simulink model "sim_IntMRE_case3"  (R2023a)
settings: Solver=ode3  StartTime=0.0  StopTime=150  FixedStep=Ts  MaxStep=Ts  RelTol=1e-4
values from neighbouring files (symbols this model uses):
  b0 = 30    [Initial_par.m]
  b1 = 11    [Initial_par.m]
  c1 = 1    [Initial_par.m]    (also in Regressor.m = c(1); virtual_ctrl.m = c(1))
  c2 = 1    [Initial_par.m]    (also in Regressor.m = c(2); virtual_ctrl.m = c(2))
  c3 = 1    [Initial_par.m]    (also in Regressor.m = c(3); virtual_ctrl.m = c(3))
  gamma = 10    [Initial_par.m]
  kpa = [kap1,kap2,kap3]    [Initial_par.m]
  N = 3    [Initial_par.m]
  tau_d = 5    [Initial_par.m]
  th = [0.4,0.5,0.1]'    [Initial_par.m]    (also in Regressor.m = th_ext(:,1); virtual_ctrl.m = th_ext(:,1))
  Ts = 1e-3    (= 0.001)    [Initial_par.m]
  vari = SD^2    (= 1e-08)    [Initial_par.m]
  x0 = [0,0,0]'    [Initial_par.m]    (also in TO_sys.m = x_init)
  zeta0 = -z0    [Initial_par.m]
undefined symbols (not defined in the file or in its folder): Phi0, z0
libraries: matrix_library x6
settings Model: Creator=stt  LastModifiedBy=stt
settings SolverCC: SolverResetMethod=Robust
settings OptimizationCC: ReuseModelBlockBuffer=off

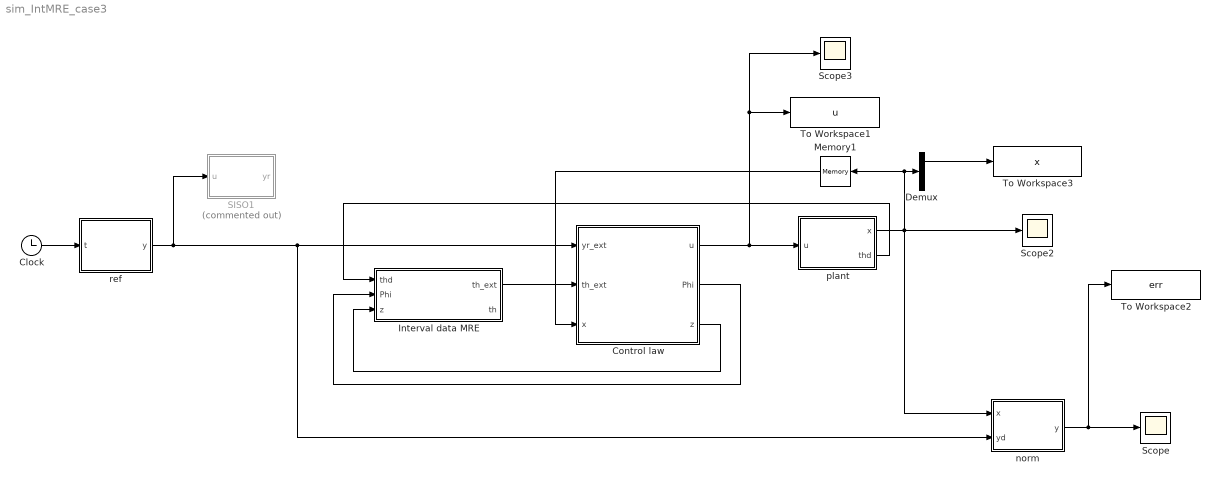
== system sim_IntMRE_case3 ==
  Clock : Clock
  Control law : Subsystem
  Demux : Demux  Outputs=3
  Interval data MRE : Subsystem
  Memory1 : Memory  InitialCondition=x0
  SISO1 : Subsystem  Commented=on
  Scope : Scope
  Scope2 : Scope
  Scope3 : Scope
  To Workspace1 : ToWorkspace  VariableName=u  SaveFormat=Timeseries  SampleTime=-1
  To Workspace2 : ToWorkspace  VariableName=err  SaveFormat=Timeseries  SampleTime=-1
  To Workspace3 : ToWorkspace  VariableName=x  SaveFormat=Timeseries  SampleTime=-1
  norm : MATLAB Function  TreatAsAtomicUnit=on
  plant : Subsystem
  ref : MATLAB Function  TreatAsAtomicUnit=on
  wires:
  ref/1(y) -> norm/2(yd), Control law/1(yr_ext), SISO1/1(u)
  norm/1(y) -> To Workspace2/1, Scope/1
  plant/1(x) -> Demux/1, Memory1/1, norm/1(x), Scope2/1
  Demux/1 -> To Workspace3/1
  Clock/1 -> ref/1(t)
  Control law/2(Phi) -> Interval data MRE/2(Phi)
  Control law/1(u) -> To Workspace1/1, Scope3/1, plant/1(u)
  Memory1/1 -> Control law/3(x)
  Interval data MRE/1(th_ext) -> Control law/2(th_ext)
  Control law/3(z) -> Interval data MRE/3(z)
  plant/2(thd) -> Interval data MRE/1(thd)

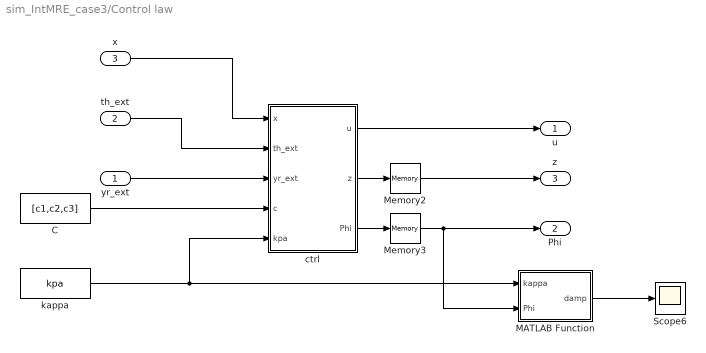
== system sim_IntMRE_case3/Control law ==
  yr_ext : Inport
  th_ext : Inport  Port=2
  x : Inport  Port=3
  C : Constant  Value=[c1,c2,c3]
  MATLAB Function : MATLAB Function  TreatAsAtomicUnit=on
  Memory2 : Memory  InitialCondition=z0
  Memory3 : Memory  InitialCondition=Phi0
  Scope6 : Scope
  ctrl : MATLAB Function  TreatAsAtomicUnit=on
  kappa : Constant  Value=kpa
  u : Outport
  Phi : Outport  Port=2
  z : Outport  Port=3
  wires:
  ctrl/3(Phi) -> Memory3/1
  Memory3/1 -> MATLAB Function/2(Phi), Phi/1
  th_ext/1 -> ctrl/2(th_ext)
  kappa/1 -> ctrl/5(kpa), MATLAB Function/1(kappa)
  C/1 -> ctrl/4(c)
  Memory2/1 -> z/1
  ctrl/2(z) -> Memory2/1
  yr_ext/1 -> ctrl/3(yr_ext)
  x/1 -> ctrl/1(x)
  ctrl/1(u) -> u/1
  MATLAB Function/1(damp) -> Scope6/1

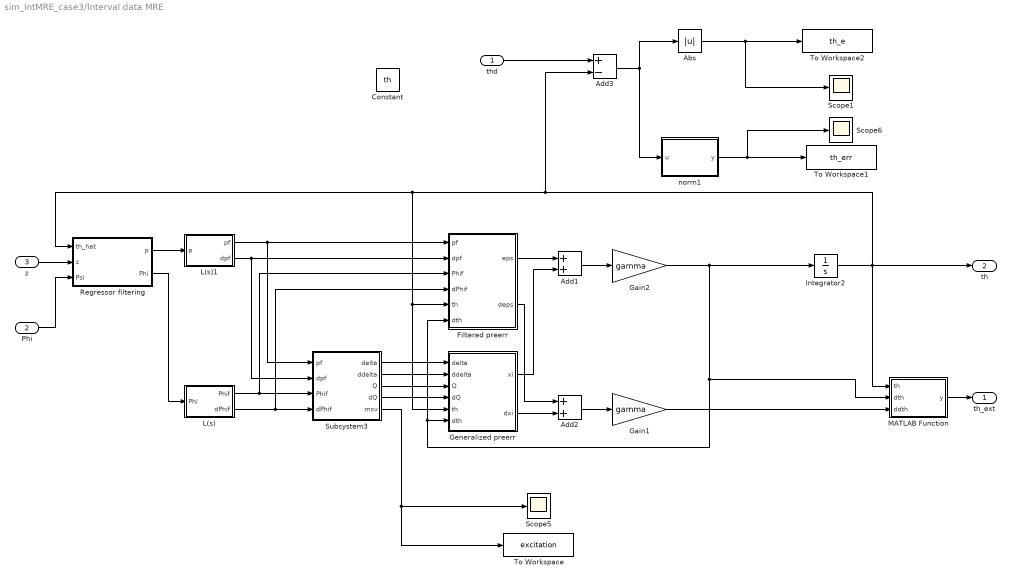
== system sim_IntMRE_case3/Interval data MRE ==
  thd : Inport
  Phi : Inport  Port=2
  z : Inport  Port=3
  Abs : Abs  SaturateOnIntegerOverflow=off
  Add1 : Sum
  Add2 : Sum
  Add3 : Sum  Inputs=+-
  Constant : Constant  Value=th
  Filtered preerr : Subsystem
  Gain1 : Gain  Gain=gamma
  Gain2 : Gain  Gain=gamma
  Generalized preerr : Subsystem
  Integrator2 : Integrator  InitialCondition=zeros(N,1)
  L(s) : Subsystem
  L(s)1 : Subsystem
  MATLAB Function : MATLAB Function  TreatAsAtomicUnit=on
  Regressor filtering : Subsystem
  Scope1 : Scope
  Scope5 : Scope
  Scope6 : Scope
  Subsystem3 : Subsystem
  To Workspace : ToWorkspace  VariableName=excitation  SaveFormat=Timeseries  SampleTime=-1
  To Workspace1 : ToWorkspace  VariableName=th_err  SaveFormat=Timeseries  SampleTime=-1
  To Workspace2 : ToWorkspace  VariableName=th_e  SaveFormat=Timeseries  SampleTime=-1
  norm1 : MATLAB Function  TreatAsAtomicUnit=on
  th_ext : Outport
  th : Outport  Port=2
  wires:
  MATLAB Function/1(y) -> th_ext/1
  norm1/1(y) -> To Workspace1/1, Scope6/1
  thd/1 -> Add3/1
  Regressor filtering/2(Phi) -> L(s)/1(Phi)
  Regressor filtering/1(p) -> L(s)1/1(p)
  z/1 -> Regressor filtering/2(z)
  Phi/1 -> Regressor filtering/3(Psi)
  Integrator2/1 -> MATLAB Function/1(th), th/1, Generalized preerr/5(th), Filtered preerr/5(th), Regressor filtering/1(th_hat), Add3/2
  Add3/1 -> norm1/1(u), Abs/1
  Abs/1 -> To Workspace2/1, Scope1/1
  L(s)1/1(pf) -> Filtered preerr/1(pf), Subsystem3/1(pf)
  L(s)1/2(dpf) -> Subsystem3/2(dpf), Filtered preerr/2(dpf)
  L(s)/1(Phif) -> Filtered preerr/3(Phif), Subsystem3/3(Phif)
  L(s)/2(dPhif) -> Filtered preerr/4(dPhif), Subsystem3/4(dPhif)
  Subsystem3/2(ddelta) -> Generalized preerr/2(ddelta)
  Subsystem3/3(Q) -> Generalized preerr/3(Q)
  Subsystem3/4(dQ) -> Generalized preerr/4(dQ)
  Subsystem3/5(msv) -> To Workspace/1, Scope5/1
  Subsystem3/1(delta) -> Generalized preerr/1(delta)
  Gain1/1 -> MATLAB Function/3(ddth)
  Add1/1 -> Gain2/1
  Filtered preerr/1(eps) -> Add1/1
  Generalized preerr/1(xi) -> Add1/2
  Generalized preerr/2(dxi) -> Add2/2
  Add2/1 -> Gain1/1
  Filtered preerr/2(deps) -> Add2/1
  Gain2/1 -> Filtered preerr/6(dth), Generalized preerr/6(dth), MATLAB Function/2(dth), Integrator2/1

== system sim_IntMRE_case3/SISO1 ==
  u : Inport
  Mux : Mux
  Scope3 : Scope
  Transfer Fcn : TransferFcn  Numerator=[16]  Denominator=[1 8 24 32 16]
  Transfer Fcn1 : TransferFcn  Numerator=[16 0]  Denominator=[1 8 24 32 16]
  Transfer Fcn2 : TransferFcn  Numerator=[16 0 0]  Denominator=[1 8 24 32 16]
  Transfer Fcn3 : TransferFcn  Numerator=[16 0 0 0]  Denominator=[1 8 24 32 16]
  yr : Outport
  wires:
  u/1 -> Transfer Fcn3/1, Transfer Fcn2/1, Transfer Fcn1/1, Transfer Fcn/1
  Transfer Fcn/1 -> Scope3/1, Mux/1
  Transfer Fcn1/1 -> Mux/2
  Transfer Fcn2/1 -> Mux/3
  Transfer Fcn3/1 -> Mux/4
  Mux/1 -> yr/1

== system sim_IntMRE_case3/plant ==
  u : Inport
  Add : Sum
  MATLAB Function : MATLAB Function  TreatAsAtomicUnit=on
  Random Number : RandomNumber  Variance=vari  SampleTime=Ts
  S-Function : S-Function  FunctionName=TO_sys  Parameters=x0,th  SFunctionDeploymentMode=off  EnableBusSupport=off
  x : Outport
  thd : Outport  Port=2
  wires:
  u/1 -> S-Function/1
  S-Function/1 -> MATLAB Function/1(u)
  Add/1 -> x/1
  MATLAB Function/2(thd) -> thd/1
  MATLAB Function/1(x) -> Add/2

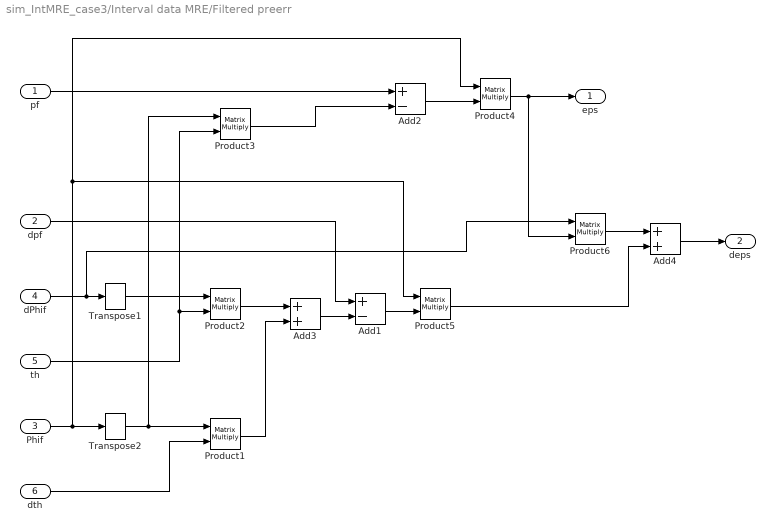
== system sim_IntMRE_case3/Interval data MRE/Filtered preerr ==
  pf : Inport
  dpf : Inport  Port=2
  Phif : Inport  Port=3
  dPhif : Inport  Port=4
  th : Inport  Port=5
  dth : Inport  Port=6
  Add1 : Sum  Inputs=+-
  Add2 : Sum  Inputs=+-
  Add3 : Sum
  Add4 : Sum
  Product{1..6} (6 alike) : Product  Multiplication=Matrix(*)
  Transpose1 : matrix_library/Transpose
  Transpose2 : matrix_library/Transpose
  eps : Outport
  deps : Outport  Port=2
  wires:
  Product2/1 -> Add3/1
  Phif/1 -> Product4/1, Product5/1, Transpose2/1
  dth/1 -> Product1/2
  Product1/1 -> Add3/2
  Add3/1 -> Add1/2
  dpf/1 -> Add1/1
  th/1 -> Product3/2, Product2/2
  Product3/1 -> Add2/2
  Transpose2/1 -> Product3/1, Product1/1
  pf/1 -> Add2/1
  Product4/1 -> Product6/2, eps/1
  Transpose1/1 -> Product2/1
  Add4/1 -> deps/1
  Add2/1 -> Product4/2
  Add1/1 -> Product5/2
  Product5/1 -> Add4/2
  dPhif/1 -> Product6/1, Transpose1/1
  Product6/1 -> Add4/1

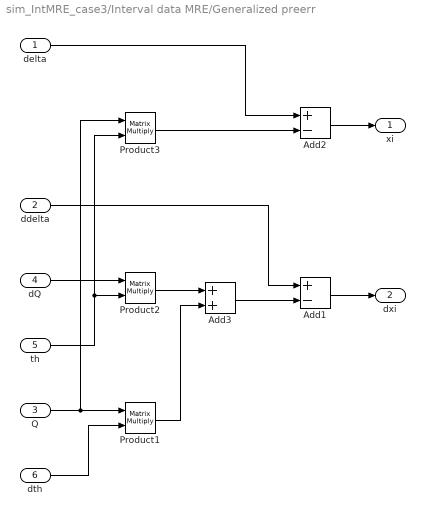
== system sim_IntMRE_case3/Interval data MRE/Generalized preerr ==
  delta : Inport
  ddelta : Inport  Port=2
  Q : Inport  Port=3
  dQ : Inport  Port=4
  th : Inport  Port=5
  dth : Inport  Port=6
  Add1 : Sum  Inputs=+-
  Add2 : Sum  Inputs=+-
  Add3 : Sum
  Product1 : Product  Multiplication=Matrix(*)
  Product2 : Product  Multiplication=Matrix(*)
  Product3 : Product  Multiplication=Matrix(*)
  xi : Outport
  dxi : Outport  Port=2
  wires:
  dQ/1 -> Product2/1
  Product2/1 -> Add3/1
  dth/1 -> Product1/2
  Product1/1 -> Add3/2
  Add3/1 -> Add1/2
  ddelta/1 -> Add1/1
  Add1/1 -> dxi/1
  th/1 -> Product3/2, Product2/2
  Product3/1 -> Add2/2
  Q/1 -> Product3/1, Product1/1
  delta/1 -> Add2/1
  Add2/1 -> xi/1

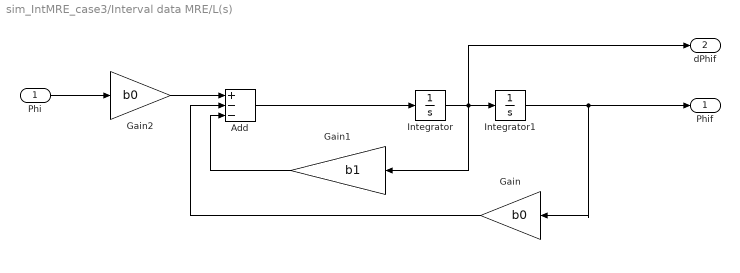
== system sim_IntMRE_case3/Interval data MRE/L(s) ==
  Phi : Inport
  Add : Sum  Inputs=+--
  Gain : Gain  Gain=b0
  Gain1 : Gain  Gain=b1
  Gain2 : Gain  Gain=b0
  Integrator : Integrator
  Integrator1 : Integrator
  Phif : Outport
  dPhif : Outport  Port=2
  wires:
  Phi/1 -> Gain2/1
  Integrator1/1 -> Gain/1, Phif/1
  Add/1 -> Integrator/1
  Integrator/1 -> Gain1/1, dPhif/1, Integrator1/1
  Gain1/1 -> Add/3
  Gain/1 -> Add/2
  Gain2/1 -> Add/1

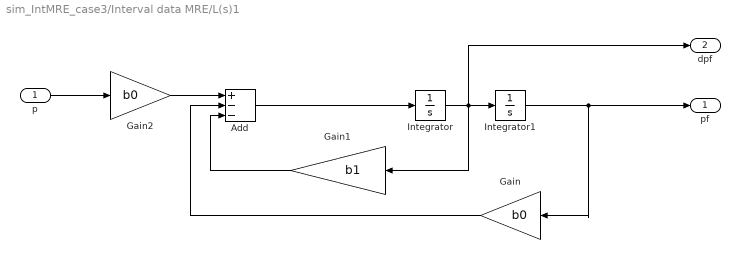
== system sim_IntMRE_case3/Interval data MRE/L(s)1 ==
  p : Inport
  Add : Sum  Inputs=+--
  Gain : Gain  Gain=b0
  Gain1 : Gain  Gain=b1
  Gain2 : Gain  Gain=b0
  Integrator : Integrator
  Integrator1 : Integrator
  pf : Outport
  dpf : Outport  Port=2
  wires:
  p/1 -> Gain2/1
  Integrator1/1 -> Gain/1, pf/1
  Add/1 -> Integrator/1
  Integrator/1 -> Gain1/1, dpf/1, Integrator1/1
  Gain1/1 -> Add/3
  Gain/1 -> Add/2
  Gain2/1 -> Add/1

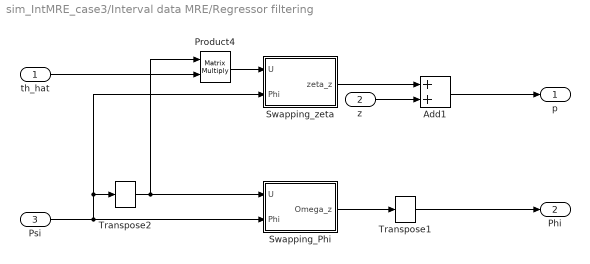
== system sim_IntMRE_case3/Interval data MRE/Regressor filtering ==
  th_hat : Inport
  z : Inport  Port=2
  Psi : Inport  Port=3
  Add1 : Sum
  Product4 : Product  Multiplication=Matrix(*)
  Swapping_Phi : Subsystem
  Swapping_zeta : Subsystem
  Transpose1 : matrix_library/Transpose
  Transpose2 : matrix_library/Transpose
  p : Outport
  Phi : Outport  Port=2
  wires:
  Product4/1 -> Swapping_zeta/1(U)
  th_hat/1 -> Product4/2
  Psi/1 -> Swapping_Phi/2(Phi), Swapping_zeta/2(Phi), Transpose2/1
  Swapping_zeta/1(zeta_z) -> Add1/1
  Transpose2/1 -> Swapping_Phi/1(U), Product4/1
  z/1 -> Add1/2
  Add1/1 -> p/1
  Swapping_Phi/1(Omega_z) -> Transpose1/1
  Transpose1/1 -> Phi/1

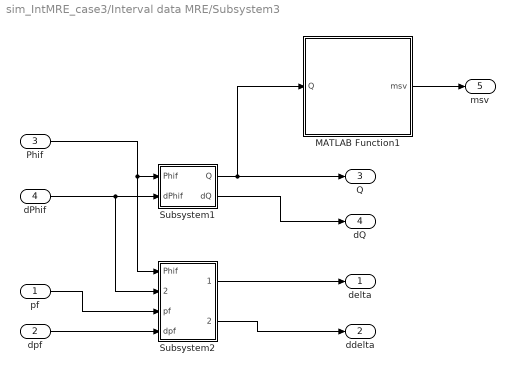
== system sim_IntMRE_case3/Interval data MRE/Subsystem3 ==
  pf : Inport
  dpf : Inport  Port=2
  Phif : Inport  Port=3
  dPhif : Inport  Port=4
  MATLAB Function1 : MATLAB Function  TreatAsAtomicUnit=on
  Subsystem1 : Subsystem
  Subsystem2 : Subsystem
  delta : Outport
  ddelta : Outport  Port=2
  Q : Outport  Port=3
  dQ : Outport  Port=4
  msv : Outport  Port=5
  wires:
  dPhif/1 -> Subsystem2/2(dPhif), Subsystem1/2(dPhif)
  Phif/1 -> Subsystem1/1(Phif), Subsystem2/1(Phif)
  pf/1 -> Subsystem2/3(pf)
  dpf/1 -> Subsystem2/4(dpf)
  MATLAB Function1/1(msv) -> msv/1
  Subsystem2/2(ddelta) -> ddelta/1
  Subsystem2/1(delta) -> delta/1
  Subsystem1/2(dQ) -> dQ/1
  Subsystem1/1(Q) -> MATLAB Function1/1(Q), Q/1

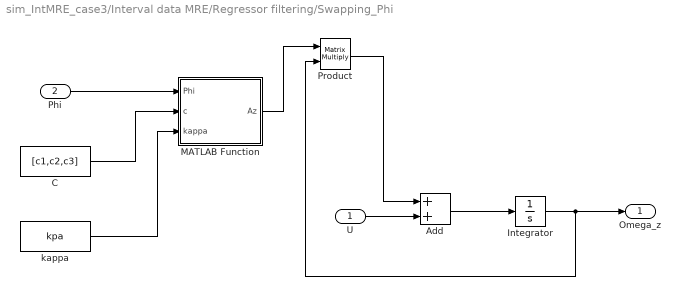
== system sim_IntMRE_case3/Interval data MRE/Regressor filtering/Swapping_Phi ==
  U : Inport
  Phi : Inport  Port=2
  Add : Sum
  C : Constant  Value=[c1,c2,c3]
  Integrator : Integrator
  MATLAB Function : MATLAB Function  TreatAsAtomicUnit=on
  Product : Product  Multiplication=Matrix(*)
  kappa : Constant  Value=kpa
  Omega_z : Outport
  wires:
  Phi/1 -> MATLAB Function/1(Phi)
  C/1 -> MATLAB Function/2(c)
  kappa/1 -> MATLAB Function/3(kappa)
  MATLAB Function/1(Az) -> Product/1
  Product/1 -> Add/1
  Add/1 -> Integrator/1
  U/1 -> Add/2
  Integrator/1 -> Product/2, Omega_z/1

== system sim_IntMRE_case3/Interval data MRE/Regressor filtering/Swapping_zeta ==
  U : Inport
  Phi : Inport  Port=2
  Add : Sum
  C : Constant  Value=[c1,c2,c3]
  Integrator : Integrator  InitialCondition=zeta0
  MATLAB Function : MATLAB Function  TreatAsAtomicUnit=on
  Product : Product  Multiplication=Matrix(*)
  kappa : Constant  Value=kpa
  zeta_z : Outport
  wires:
  Phi/1 -> MATLAB Function/1(Phi)
  C/1 -> MATLAB Function/2(c)
  kappa/1 -> MATLAB Function/3(kappa)
  MATLAB Function/1(Az) -> Product/1
  Product/1 -> Add/1
  Add/1 -> Integrator/1
  U/1 -> Add/2
  Integrator/1 -> Product/2, zeta_z/1

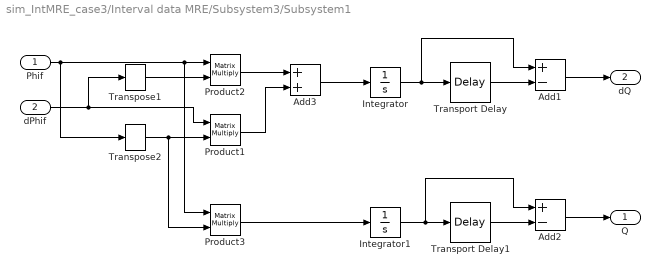
== system sim_IntMRE_case3/Interval data MRE/Subsystem3/Subsystem1 ==
  Phif : Inport
  dPhif : Inport  Port=2
  Add1 : Sum  Inputs=+-
  Add2 : Sum  Inputs=+-
  Add3 : Sum
  Integrator : Integrator
  Integrator1 : Integrator
  Product1 : Product  Multiplication=Matrix(*)
  Product2 : Product  Multiplication=Matrix(*)
  Product3 : Product  Multiplication=Matrix(*)
  Transport Delay : TransportDelay  DelayTime=tau_d
  Transport Delay1 : TransportDelay  DelayTime=tau_d
  Transpose1 : matrix_library/Transpose
  Transpose2 : matrix_library/Transpose
  Q : Outport
  dQ : Outport  Port=2
  wires:
  Phif/1 -> Product3/1, Product2/1, Transpose2/1
  dPhif/1 -> Product1/1, Transpose1/1
  Product1/1 -> Add3/2
  Transpose1/1 -> Product2/2
  Transpose2/1 -> Product3/2, Product1/2
  Product2/1 -> Add3/1
  Add3/1 -> Integrator/1
  Integrator/1 -> Add1/1, Transport Delay/1
  Transport Delay/1 -> Add1/2
  Add1/1 -> dQ/1
  Product3/1 -> Integrator1/1
  Transport Delay1/1 -> Add2/2
  Integrator1/1 -> Transport Delay1/1, Add2/1
  Add2/1 -> Q/1

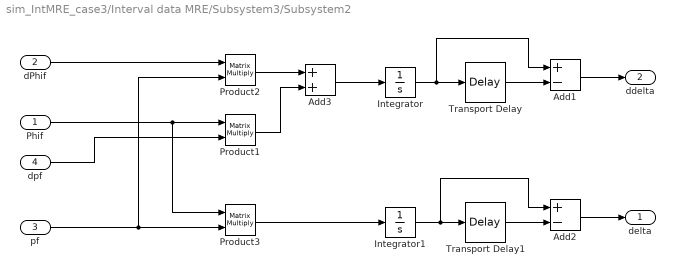
== system sim_IntMRE_case3/Interval data MRE/Subsystem3/Subsystem2 ==
  Phif : Inport
  dPhif : Inport  Port=2
  pf : Inport  Port=3
  dpf : Inport  Port=4
  Add1 : Sum  Inputs=+-
  Add2 : Sum  Inputs=+-
  Add3 : Sum
  Integrator : Integrator
  Integrator1 : Integrator
  Product1 : Product  Multiplication=Matrix(*)
  Product2 : Product  Multiplication=Matrix(*)
  Product3 : Product  Multiplication=Matrix(*)
  Transport Delay : TransportDelay  DelayTime=tau_d
  Transport Delay1 : TransportDelay  DelayTime=tau_d
  delta : Outport
  ddelta : Outport  Port=2
  wires:
  Product3/1 -> Integrator1/1
  Add1/1 -> ddelta/1
  Transport Delay/1 -> Add1/2
  Integrator/1 -> Add1/1, Transport Delay/1
  Transport Delay1/1 -> Add2/2
  Add2/1 -> delta/1
  Add3/1 -> Integrator/1
  Integrator1/1 -> Transport Delay1/1, Add2/1
  Product1/1 -> Add3/2
  Product2/1 -> Add3/1
  dPhif/1 -> Product2/1
  pf/1 -> Product2/2, Product3/2
  Phif/1 -> Product3/1, Product1/1
  dpf/1 -> Product1/2

== matlab function sim_IntMRE_case3/Control law/ctrl ==
  data: x input; th_ext input; yr_ext input; u output; c input; kpa input; z output; Phi output
function [u,z,Phi] = fcn(x,th_ext,yr_ext,c,kpa)



[alpha1,alpha2,u,z,Phi]=virtual_ctrl(x,th_ext,yr_ext,kpa,c);
vir_u=[alpha1,alpha2];

== matlab function sim_IntMRE_case3/Interval data MRE/Subsystem3/MATLAB Function1 ==
  data: Q input; msv output
function msv = fcn(Q)

msv = min(svd(Q));

== matlab function sim_IntMRE_case3/ref ==
  data: t input; y output
function y = fcn(t)

% if t<10
%     y=1;
% % elseif t<80
%     % y=-0.5;
% elseif t<60
%     y=0.5;
% else
%     y=-1;
% end


A=1;T=1;
y=[A*sin(T*t);A*T*cos(T*t);-A*T*T*sin(T*t);-A*T*T*T*cos(T*t)];
% y=1.2*sin(0.8*t)+0.8*cos(0.4*t)-0.8;

== matlab function sim_IntMRE_case3/norm ==
  data: x input; y output; yd input
function y= fcn(x,yd)
err=x(1)-yd(1);
y = abs(err);

== matlab function sim_IntMRE_case3/Interval data MRE/Regressor filtering/Swapping_zeta/MATLAB Function ==
  data: Phi input; Az output; c input; kappa input
function Az = fcn(Phi,c,kappa)
c1=c(1);c2=c(2);c3=c(3);
kap1=kappa(1);kap2=kappa(2);kap3=kappa(3);
phi1=Phi(:,1);phi2=Phi(:,2);phi3=Phi(:,3);
Dg=-[c1+kap1*norm(phi1)^2,c2+kap2*norm(phi2)^2,c3+kap3*norm(phi3)^2];
Az=diag(Dg)+diag([1,1],1)-diag([1,1],-1);

== matlab function sim_IntMRE_case3/Interval data MRE/Regressor filtering/Swapping_Phi/MATLAB Function ==
  data: Phi input; Az output; c input; kappa input
function Az = fcn(Phi,c,kappa)
c1=c(1);c2=c(2);c3=c(3);
kap1=kappa(1);kap2=kappa(2);kap3=kappa(3);
phi1=Phi(:,1);phi2=Phi(:,2);phi3=Phi(:,3);
Dg=-[c1+kap1*norm(phi1)^2,c2+kap2*norm(phi2)^2,c3+kap3*norm(phi3)^2];
Az=diag(Dg)+diag([1,1],1)-diag([1,1],-1);

== matlab function sim_IntMRE_case3/plant/MATLAB Function ==
  data: u input; x output; thd output
function [x,thd] = fcn(u)

x=u(1:3);
thd=u(4:6);

== matlab function sim_IntMRE_case3/Interval data MRE/MATLAB Function ==
  data: th input; y output; dth input; ddth input
function y = fcn(th,dth,ddth)

y = [th,dth,ddth];

== matlab function sim_IntMRE_case3/Interval data MRE/norm1 ==
  data: u input; y output
function y = fcn(u)

y = norm(u);

== matlab function sim_IntMRE_case3/Control law/MATLAB Function ==
  data: kappa input; damp output; Phi input
function damp = fcn(kappa,Phi)
kap1=kappa(1);kap2=kappa(2);kap3=kappa(3);
phi1=Phi(:,1);phi2=Phi(:,2);phi3=Phi(:,3);
damp=-[kap1*norm(phi1)^2,kap2*norm(phi2)^2,kap3*norm(phi3)^2];
